simulink model "EstimadorComAtrasoGammaChaveado"  (R2015a)
settings: Solver=ode45  StartTime=0.0  StopTime=200  RelTol=1e-3
settings Model: Creator=user  LastModifiedBy=user
settings SolverCC: ZeroCrossControl=DisableAll

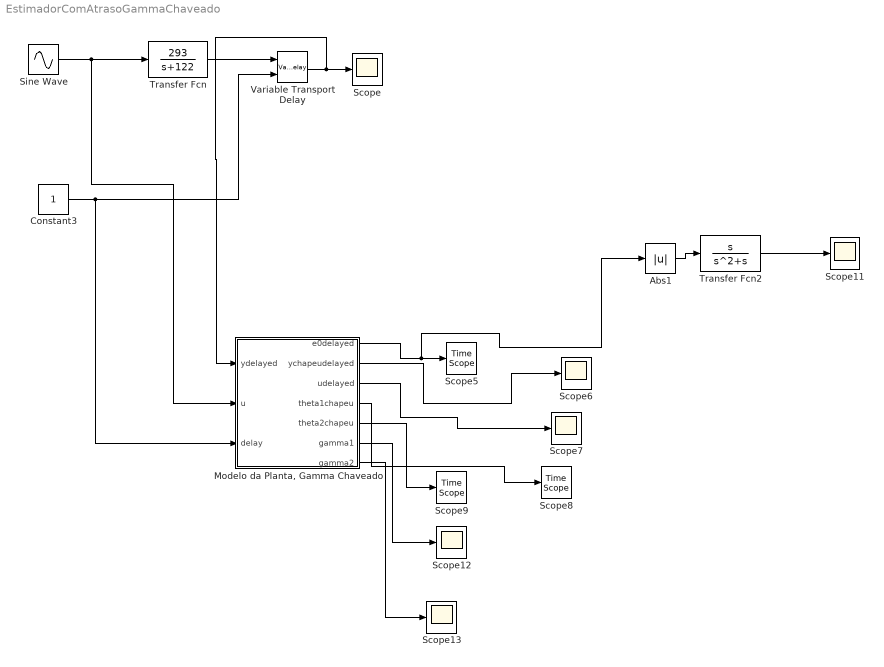
== system EstimadorComAtrasoGammaChaveado ==
  Abs1 : Abs
  Constant3 : Constant
  "Modelo da Planta, Gamma Chaveado" : Subsystem  Description=First Order Transfer Function Estimation Block
  Scope{,6..7,11..13} (6 alike) : Scope
      Scope11 settings: YMin=-3.46945e-18  YMax=0.14  SaveName=ScopeData11
      Scope12 settings: YMin=1  YMax=1  SaveName=ScopeData12
      Scope13 settings: YMin=111  YMax=111  SaveName=ScopeData13
      Scope6 settings: YMin=-0.35  YMax=0.3  SaveName=ScopeData6
      Scope7 settings: YMin=-1  YMax=1  SaveName=ScopeData7
  Scope5 : TimeScope
  Scope8 : TimeScope
  Scope9 : TimeScope
  Sine Wave : Sin  Frequency=10  SampleTime=0
  Transfer Fcn : TransferFcn  Numerator=[293]  Denominator=[1 122]
  Transfer Fcn2 : TransferFcn  Numerator=[1 0]  Denominator=[1 1 0]
  Variable Transport Delay : VariableTransportDelay  VariableDelayType=Variable transport delay  MaximumDelay=10  MaximumPoints=4096
  wires:
  Sine Wave/1 -> "Modelo da Planta, Gamma Chaveado"/2(u), Transfer Fcn/1
  Transfer Fcn/1 -> Variable Transport Delay/1
  Variable Transport Delay/1 -> "Modelo da Planta, Gamma Chaveado"/1(ydelayed), Scope/1
  "Modelo da Planta, Gamma Chaveado"/2(ychapeudelayed) -> Scope6/1
  "Modelo da Planta, Gamma Chaveado"/3(udelayed) -> Scope7/1
  "Modelo da Planta, Gamma Chaveado"/4(theta1chapeu) -> Scope8/1
  "Modelo da Planta, Gamma Chaveado"/5(theta2chapeu) -> Scope9/1
  "Modelo da Planta, Gamma Chaveado"/1(e0delayed) -> Abs1/1, Scope5/1
  Transfer Fcn2/1 -> Scope11/1
  Abs1/1 -> Transfer Fcn2/1
  "Modelo da Planta, Gamma Chaveado"/6(gamma1) -> Scope12/1
  "Modelo da Planta, Gamma Chaveado"/7(gamma2) -> Scope13/1
  Constant3/1 -> "Modelo da Planta, Gamma Chaveado"/3(delay), Variable Transport Delay/2

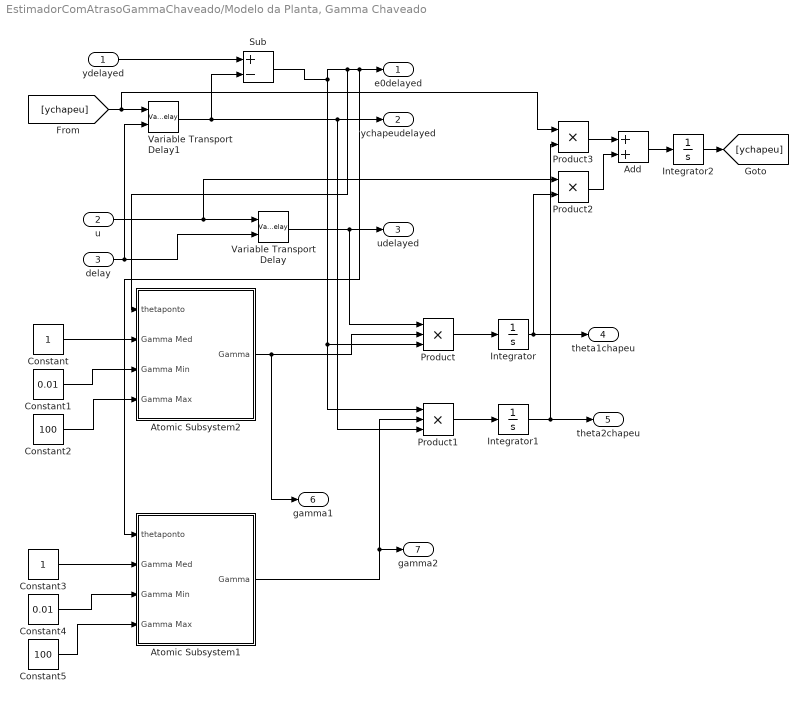
== system EstimadorComAtrasoGammaChaveado/Modelo da Planta, Gamma Chaveado ==
  ydelayed : Inport
  u : Inport  Port=2
  delay : Inport  Port=3
  Add : Sum
  Atomic Subsystem1 : Subsystem  TreatAsAtomicUnit=on
  Atomic Subsystem2 : Subsystem  TreatAsAtomicUnit=on
  Constant : Constant
  Constant1 : Constant  Value=0.01
  Constant2 : Constant  Value=100
  Constant3 : Constant
  Constant4 : Constant  Value=0.01
  Constant5 : Constant  Value=100
  Integrator : Integrator
  Integrator1 : Integrator
  Integrator2 : Integrator
  Product : Product  Inputs=3
  Product1 : Product  Inputs=3
  Product2 : Product
  Product3 : Product
  Sub : Sum  Inputs=+-
  Variable Transport Delay : VariableTransportDelay  VariableDelayType=Variable transport delay  MaximumDelay=10
  Variable Transport Delay1 : VariableTransportDelay  VariableDelayType=Variable transport delay  MaximumDelay=10
  e0delayed : Outport
  ychapeudelayed : Outport  Port=2
  udelayed : Outport  Port=3
  theta1chapeu : Outport  Port=4
  theta2chapeu : Outport  Port=5
  gamma1 : Outport  Port=6
  gamma2 : Outport  Port=7
  wires:
  ydelayed/1 -> Sub/1
  delay/1 -> Variable Transport Delay1/2, Variable Transport Delay/2
  u/1 -> Product2/1, Variable Transport Delay/1
  Variable Transport Delay/1 -> Product/1, udelayed/1
  Atomic Subsystem2/1(Gamma) -> gamma1/1, Product/2
  Product/1 -> Integrator/1
  Integrator/1 -> Product2/2, theta1chapeu/1
  Atomic Subsystem1/1(Gamma) -> gamma2/1, Product1/2
  [ychapeu] -> Product3/1, Variable Transport Delay1/1
  Variable Transport Delay1/1 -> Product1/3, ychapeudelayed/1, Sub/2
  Product1/1 -> Integrator1/1
  Integrator1/1 -> Product3/2, theta2chapeu/1
  Product3/1 -> Add/1
  Product2/1 -> Add/2
  Add/1 -> Integrator2/1
  Integrator2/1 -> [ychapeu]
  Constant/1 -> Atomic Subsystem2/2(Gamma Med)
  Constant1/1 -> Atomic Subsystem2/3(Gamma Min)
  Constant2/1 -> Atomic Subsystem2/4(Gamma Max)
  Constant3/1 -> Atomic Subsystem1/2(Gamma Med)
  Constant4/1 -> Atomic Subsystem1/3(Gamma Min)
  Constant5/1 -> Atomic Subsystem1/4(Gamma Max)
  Sub/1 -> Product1/1, Product/3, Atomic Subsystem2/1(thetaponto), Atomic Subsystem1/1(thetaponto), e0delayed/1

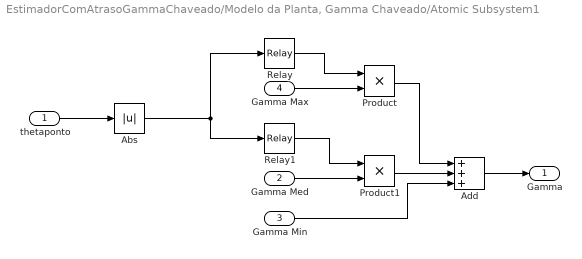
== system EstimadorComAtrasoGammaChaveado/Modelo da Planta, Gamma Chaveado/Atomic Subsystem1 ==
  thetaponto : Inport
  Gamma Med : Inport  Port=2
  Gamma Min : Inport  Port=3
  Gamma Max : Inport  Port=4
  Abs : Abs
  Add : Sum  Inputs=+++
  Product : Product
  Product1 : Product
  Relay : Relay  OnSwitchValue=0.01  OffSwitchValue=0.01  OnOutputValue=0  OffOutputValue=1
  Relay1 : Relay  OnSwitchValue=0.1  OffSwitchValue=0.1  OnOutputValue=0  OffOutputValue=1
  Gamma : Outport
  wires:
  thetaponto/1 -> Abs/1
  Gamma Max/1 -> Product/2
  Relay/1 -> Product/1
  Gamma Med/1 -> Product1/2
  Relay1/1 -> Product1/1
  Product/1 -> Add/1
  Product1/1 -> Add/2
  Gamma Min/1 -> Add/3
  Add/1 -> Gamma/1
  Abs/1 -> Relay1/1, Relay/1

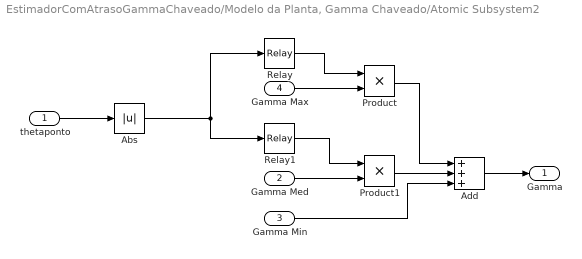
== system EstimadorComAtrasoGammaChaveado/Modelo da Planta, Gamma Chaveado/Atomic Subsystem2 ==
  thetaponto : Inport
  Gamma Med : Inport  Port=2
  Gamma Min : Inport  Port=3
  Gamma Max : Inport  Port=4
  Abs : Abs
  Add : Sum  Inputs=+++
  Product : Product
  Product1 : Product
  Relay : Relay  OnSwitchValue=0.01  OffSwitchValue=0.01  OnOutputValue=0  OffOutputValue=1
  Relay1 : Relay  OnSwitchValue=0.1  OffSwitchValue=0.1  OnOutputValue=0  OffOutputValue=1
  Gamma : Outport
  wires:
  thetaponto/1 -> Abs/1
  Gamma Max/1 -> Product/2
  Relay/1 -> Product/1
  Gamma Med/1 -> Product1/2
  Relay1/1 -> Product1/1
  Product/1 -> Add/1
  Product1/1 -> Add/2
  Gamma Min/1 -> Add/3
  Add/1 -> Gamma/1
  Abs/1 -> Relay1/1, Relay/1
